simulink model "VehicleDynamicsModel"  (R2018a)
settings: Solver=ode15s  StartTime=0.0  StopTime=12  FixedStep=0.01  RelTol=1e-2  EnableMultiTasking=on
PreLoadFcn:
  | PowerTrain_14DOF_ini
StopFcn:
  | AfterSim
undefined symbols (not defined in the file): AccelCmd2TrqCmd, Chasis, GearRatio, Motor, Motor_J, Motor_RotorDamping, VEH, X, Y, Z
libraries: sm_lib x186, autolibutils x40, nesl_utility x23, vehdynlibtire x4, fuzblock x3, sharedtransform x2, autolibmappedmotorcommon x2, vehdynlibeom x1, vehdynlibsuspension x1, simulink x1, vehdynlibsteering x1
(part 4 of 11)

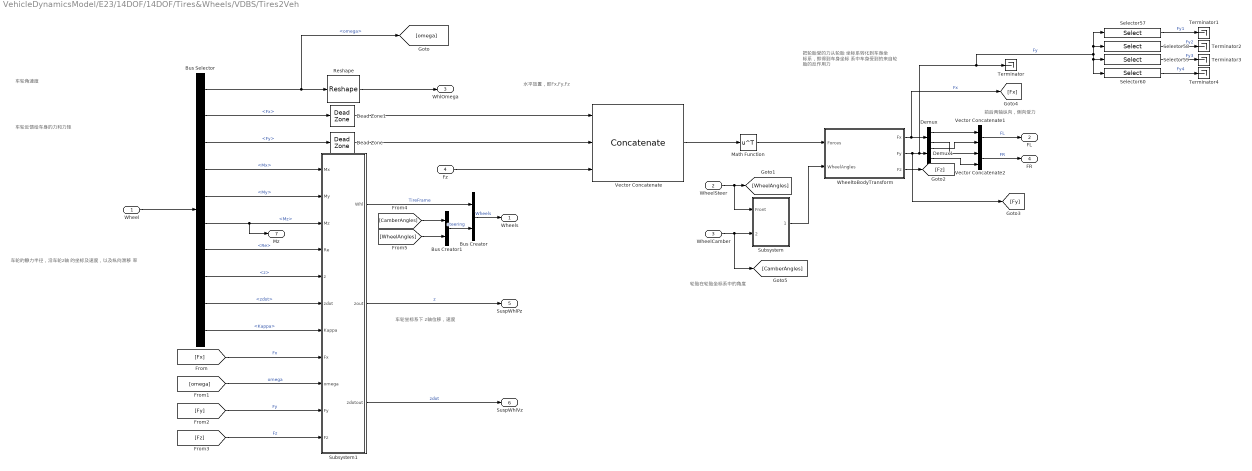
== system VehicleDynamicsModel/E23/14DOF/14DOF/Tires&Wheels/VDBS/Tires2Veh ==
  note: 车轮坐标系下
      | z轴位移，速度
  note: 水平放置，即Fx,Fy,Fz
  note: 轮胎在轮胎坐标系中的角度
  note: 车轮角速度
  note: 车轮的静力半径，沿车轮z轴
      | 的坐标及速度，以及纵向滑移
      | 率
  note: 车轮反馈给车身的力和力矩
  note: 前后两轴纵向，侧向受力
  note: 把轮胎受的力从轮胎
      | 坐标系转化到车身坐
      | 标系，即得到车身坐标
      | 系中车身受到的来自轮
      | 胎的反作用力
  Wheel : Inport
  WheelSteer : Inport  Port=2
  WheelCamber : Inport  Port=3
  Fz : Inport  Port=4
  Bus Creator : BusCreator  Inputs=2
  Bus Creator1 : BusCreator  Inputs=2
  Bus Selector : BusSelector  OutputSignals=omega,Fx,Fy,Mx,My,Mz,Re,z,zdot,Kappa
  Dead Zone : DeadZone  LowerValue=-10  UpperValue=10  SaturateOnIntegerOverflow=on
  Dead Zone1 : DeadZone  LowerValue=-5  UpperValue=5  SaturateOnIntegerOverflow=on
  Demux : Demux  Outputs=2
  Demux1 : Demux  Outputs=2
  Math Function : Math  Operator=transpose  SaturateOnIntegerOverflow=on
  Reshape : Reshape  OutputDimensionality=Customize  OutputDimensions=[2,2]
  Selector57 : Selector  InputPortWidth=4  IndexOptions=Index vector (dialog)  Indices=1  OutputSizes=1
  Selector58 : Selector  InputPortWidth=4  IndexOptions=Index vector (dialog)  Indices=2  OutputSizes=1
  Selector59 : Selector  InputPortWidth=4  IndexOptions=Index vector (dialog)  Indices=3  OutputSizes=1
  Selector60 : Selector  InputPortWidth=4  IndexOptions=Index vector (dialog)  Indices=4  OutputSizes=1
  Subsystem : Subsystem
  Subsystem1 : Subsystem
  Terminator{,1..4} (5 alike) : Terminator
  Vector Concatenate : Concatenate  NumInputs=3  Mode=Multidimensional array  ConcatenateDimension=2
  Vector Concatenate1 : Concatenate  Mode=Multidimensional array
  Vector Concatenate2 : Concatenate  Mode=Multidimensional array
  WheeltoBodyTransform : Subsystem  TreatAsAtomicUnit=on
  Wheels : Outport
  FL : Outport  Port=2
  "WhlOmega " : Outport  Port=3
  FR : Outport  Port=4
  SuspWhlPz : Outport  Port=5
  SuspWhlVz : Outport  Port=6
  Mz : Outport  Port=7
  wires:
  Wheel/1 -> Bus Selector/1
  Bus Selector/1 -> [omega], Reshape/1  "<omega>"
  Reshape/1 -> "WhlOmega "/1
  Bus Selector/2 -> Dead Zone1/1  "<Fx>"
  Bus Selector/3 -> Dead Zone/1  "<Fy>"
  Dead Zone1/1 -> Vector Concatenate/1
  Dead Zone/1 -> Vector Concatenate/2
  Fz/1 -> Vector Concatenate/3
  Vector Concatenate/1 -> Math Function/1
  Math Function/1 -> WheeltoBodyTransform/1(Forces)
  WheelSteer/1 -> Subsystem/1(Front), [WheelAngles]
  WheelCamber/1 -> [CamberAngles], Subsystem/2(Camber)
  Subsystem/1(Vehicle) -> WheeltoBodyTransform/2(WheelAngles)
  WheeltoBodyTransform/3(Fz) -> [Fz]
  WheeltoBodyTransform/1(Fx) -> [Fx], Demux/1  "Fx"
  WheeltoBodyTransform/2(Fy) -> Selector60/1, Selector59/1, Selector57/1, Selector58/1, Terminator/1, Demux1/1, [Fy]  "Fy"
  Demux/1 -> Vector Concatenate1/1
  Demux1/1 -> Vector Concatenate1/2
  Demux/2 -> Vector Concatenate2/1
  Demux1/2 -> Vector Concatenate2/2
  Vector Concatenate1/1 -> FL/1  "FL"
  Vector Concatenate2/1 -> FR/1  "FR"
  Bus Selector/4 -> Subsystem1/1(Mx)  "<Mx>"
  Bus Selector/5 -> Subsystem1/2(My)  "<My>"
  Bus Selector/6 -> Mz/1, Subsystem1/3(Mz)  "<Mz>"
  Bus Selector/7 -> Subsystem1/4(Re)  "<Re>"
  Bus Selector/8 -> Subsystem1/5(z)  "<z>"
  Bus Selector/9 -> Subsystem1/6(zdot)  "<zdot>"
  Bus Selector/10 -> Subsystem1/7(Kappa)  "<Kappa>"
  [omega] -> Subsystem1/9(omega)  "omega"
  [Fz] -> Subsystem1/11(Fz)  "Fz"
  Subsystem1/1(Whl) -> Bus Creator/1  "TireFrame"
  Bus Creator1/1 -> Bus Creator/2  "steering"
  [CamberAngles] -> Bus Creator1/1
  [WheelAngles] -> Bus Creator1/2
  Bus Creator/1 -> Wheels/1  "Wheels"
  Subsystem1/2(zout) -> SuspWhlPz/1  "z"
  Subsystem1/3(zdotout) -> SuspWhlVz/1  "zdot"
  [Fy] -> Subsystem1/10(Fy)  "Fy"
  [Fx] -> Subsystem1/8(Fx)  "Fx"
  Selector57/1 -> Terminator1/1  "Fy1"
  Selector60/1 -> Terminator4/1  "Fy4"
  Selector59/1 -> Terminator3/1  "Fy3"
  Selector58/1 -> Terminator2/1  "Fy2"

== system VehicleDynamicsModel/E23/14DOF/14DOF/Tires&Wheels/VDBS/Veh2Tire ==
  note: 为什么取反？
  note: 车轮坐标系
  r : Inport
  Axle : Inport  Port=2
  Braker : Inport  Port=3
  Camber : Inport  Port=4
  Steer : Inport  Port=5
  VelVeh : Inport  Port=6
  Demux : Demux
  Gain : Gain  Gain=[1;-1;1;-1]*0+1
  Mux : Mux
  Reshape : Reshape
  Reshape1 : Reshape
  Unary Minus : UnaryMinus
  WheelAngles : Subsystem
  WheeltoBodyTransform : Subsystem  TreatAsAtomicUnit=on
  T : Outport
  P : Outport  Port=2
  psidot : Outport  Port=3
  xdotAxle : Outport  Port=4
  ydotAxle : Outport  Port=5
  zdotAxle : Outport  Port=6
  wires:
  Braker/1 -> Reshape1/1
  Axle/1 -> Reshape/1
  Reshape1/1 -> Demux/1
  Gain/1 -> T/1  "Nm"
  Reshape/1 -> Gain/1
  Mux/1 -> P/1  "Pa"
  Demux/1 -> Mux/1
  Demux/3 -> Mux/3
  Camber/1 -> WheelAngles/1(Camber)
  Demux/2 -> Mux/2
  r/1 -> Unary Minus/1
  Demux/4 -> Mux/4
  VelVeh/1 -> WheeltoBodyTransform/2(VelVeh)
  Unary Minus/1 -> psidot/1  "RPS"
  WheeltoBodyTransform/1(xdotWheel) -> xdotAxle/1
  WheelAngles/1(Vehicle) -> WheeltoBodyTransform/1(WheelAngles)
  WheeltoBodyTransform/3(zdotWheel) -> zdotAxle/1
  WheeltoBodyTransform/2(ydotWheel) -> ydotAxle/1
  Steer/1 -> WheelAngles/2(Steer)

== system VehicleDynamicsModel/E23/14DOF/14DOF/Tires&Wheels/VDBS/scale factors with friction1 ==
  lamda_mu_x : Inport
  lamda_mu_y : Inport  Port=2
  Reshape : Reshape  OutputDimensionality=Row vector (2-D)  OutputDimensions=[1,numWheels]
  Reshape1 : Reshape  OutputDimensionality=Row vector (2-D)  OutputDimensions=[1,numWheels]
  Signal Specification : SignalSpecification  Unit=1
  Signal Specification1 : SignalSpecification  Unit=1
  Vector Concatenate : Concatenate  NumInputs=4  Mode=Multidimensional array
  ones1 : Constant  Value=[ones(24,numWheels)]  VectorParams1D=off
  ones2 : Constant  Value=ones(1,numWheels)  VectorParams1D=off
  lambdas : Outport  Unit=1
  wires:
  Reshape1/1 -> Vector Concatenate/3
  Reshape/1 -> Vector Concatenate/2
  lamda_mu_y/1 -> Reshape1/1
  lamda_mu_x/1 -> Reshape/1
  ones1/1 -> Signal Specification1/1
  ones2/1 -> Signal Specification/1
  Vector Concatenate/1 -> lambdas/1
  Signal Specification/1 -> Vector Concatenate/1
  Signal Specification1/1 -> Vector Concatenate/4
